simulink model "Signal3"  (Simulink 9.1)
settings: Solver=ode45  StartTime=0.0  StopTime=20  RelTol=1e-3  EnableMultiTasking=on
settings Model: Creator=Admin  LastModifiedBy=Asus
settings DataIOCC: LimitDataPoints=on  SignalLoggingSaveFormat=ModelDataLogs
settings OptimizationCC: ExpressionDepthLimit=2147483647
settings DebuggingCC: SolverPrmCheckMsg=warning  FcnCallInpInsideContextMsg=warning  StateNameClashWarn=warning
settings GRTTargetCC: GeneratePreprocessorConditionals=Disable all  CombineOutputUpdateFcns=on  GRTInterface=off

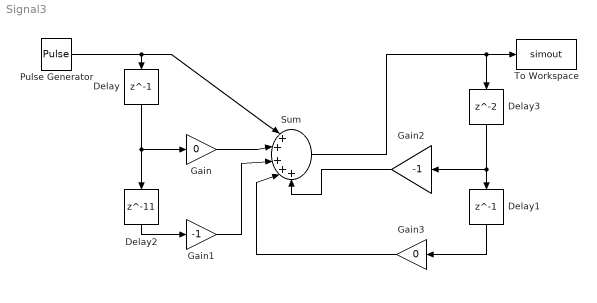
== system Signal3 ==
  Delay : Delay  DelayLength=1
  Delay1 : Delay  DelayLength=1
  Delay2 : Delay  DelayLength=11
  Delay3 : Delay
  Gain : Gain  Gain=0
  Gain1 : Gain  Gain=-1
  Gain2 : Gain  Gain=-1
  Gain3 : Gain  Gain=0
  Pulse Generator : DiscretePulseGenerator  Period=100
  Sum : Sum  Inputs=|+++++
  To Workspace : ToWorkspace  VariableName=simout  SampleTime=-1
  wires:
  Pulse Generator/1 -> Sum/1, Delay/1
  Delay/1 -> Gain/1, Delay2/1
  Delay2/1 -> Gain1/1
  Delay1/1 -> Gain3/1
  Gain1/1 -> Sum/3
  Gain/1 -> Sum/2
  Gain3/1 -> Sum/4
  Gain2/1 -> Sum/5
  Delay3/1 -> Gain2/1, Delay1/1
  Sum/1 -> To Workspace/1, Delay3/1
